simulink model "vehicle_dynamics"  (R2023a)
settings: Solver=FixedStepAuto  StartTime=0.0  StopTime=10.0  MaxStep=1e-3  RelTol=1e-3  EnableMultiTasking=on
undefined symbols (not defined in the file): A, b_vkm, c_W, eta, f_R, g, iD_car, iG_car, m_F, m_vkm, m_Zu, p, p_L, r_dyn, r_stat, v_0
settings Model: Creator=Sascha  LastModifiedBy=Sascha
settings SolverCC: AlgebraicLoopSolver=TrustRegion
settings OptimizationCC: EnhancedBackFolding=on  PassReuseOutputArgsAs=Individual arguments  ZeroExternalMemoryAtStartup=off  ZeroInternalMemoryAtStartup=off  MaxStackSize=64  OptimizeBlockOrder=speed  DifferentSizesBufferReuse=on  OptimizationCustomize=off  EfficientTunableParamExpr=on
settings DebuggingCC: ParameterTunabilityLossMsg=error  UnconnectedInputMsg=warning  UnconnectedOutputMsg=warning  UnconnectedLineMsg=warning
settings HardwareCC: ProdBitPerPointer=32  ProdBitPerSizeT=32  ProdBitPerPtrDiffT=32  ProdLargestAtomicInteger=Long  ProdLargestAtomicFloat=Double  ProdWordSize=32  ProdLongLongMode=on  ProdHWDeviceType=ARM Compatible->ARM Cortex
settings ModelReferenceCC: EnableRefExpFcnMdlSchedulingChecks=on
settings SFSimCC: MATLABDynamicMemAlloc=off
settings RTWCC: Description=Embedded Coder  SystemTargetFile=ert.tlc  HardwareBoard=STM32F746G-Discovery  TemplateMakefile=ert_default_tmf  Toolchain=GNU Tools for ARM Embedded Processors  DLArmComputeVersion=19.05
settings CodeAppCC: ForceParamTrailComments=on  IgnoreCustomStorageClasses=off  OperatorAnnotations=on  SimulinkDataObjDesc=on  SFDataObjDesc=on  InsertBlockDesc=on
settings ERTTargetCC: ExtModeTransport=3  ExtModeStaticAlloc=on  ExtModeStaticAllocSize=5000  ExtModeMexFile=ext_xcp  ExtModeIntrfLevel=Level2 - Open

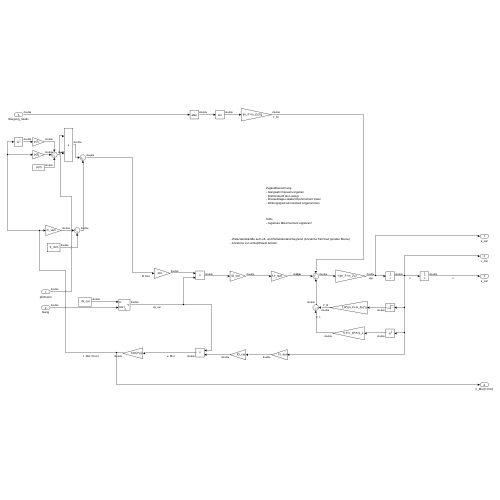
[thumbnail: Simulink's stored preview of the top-level diagram]
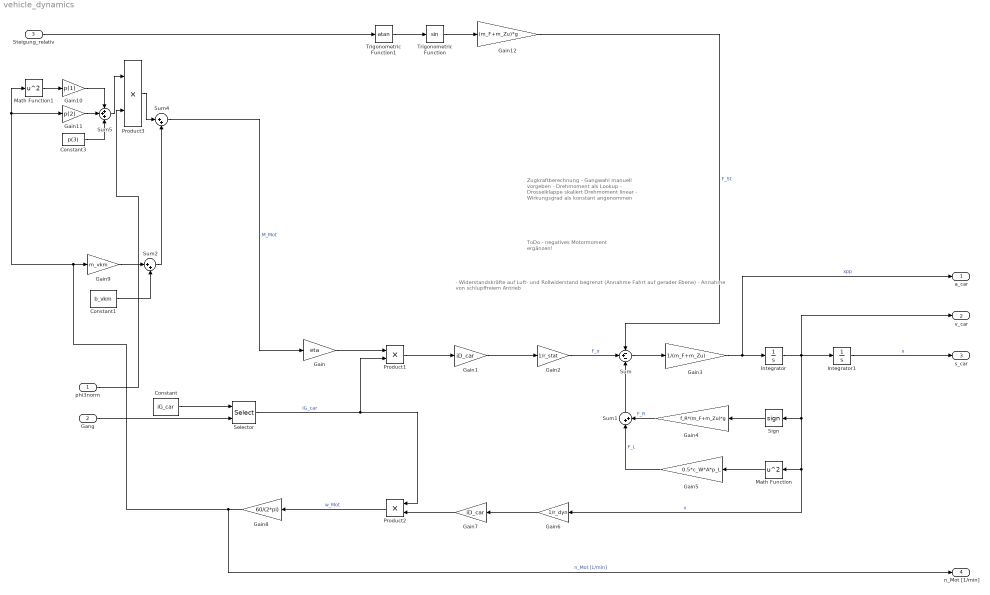
== system vehicle_dynamics ==
  note: Zugkraftberechnung
      | - Gangwahl manuell vorgeben
      | - Drehmoment als Lookup
      | - Drosselklappe skaliert Drehmoment linear
      | - Wirkungsgrad als konstant angenommen
  note: ToDo
      | - negatives Motormoment ergänzen!
  note: - Widerstandskräfte auf Luft- und Rollwiderstand begrenzt (Annahme Fahrt auf gerader Ebene)
      | - Annahme von schlupffreiem Antrieb
  phi3norm : Inport
  Gang : Inport  Port=2
  Steigung_relativ : Inport  Port=3
  Constant : Constant  Value=iG_car
  Constant1 : Constant  Value=b_vkm
  Constant3 : Constant  Value=p(3)
  Gain : Gain  Gain=eta
  Gain1 : Gain  Gain=iD_car
  Gain10 : Gain  Gain=p(1)
  Gain11 : Gain  Gain=p(2)
  Gain12 : Gain  Gain=(m_F+m_Zu)*g
  Gain2 : Gain  Gain=1/r_stat
  Gain3 : Gain  Gain=1/(m_F+m_Zu)
  Gain4 : Gain  Gain=f_R*(m_F+m_Zu)*g
  Gain5 : Gain  Gain=0.5*c_W*A*p_L
  Gain6 : Gain  Gain=1/r_dyn
  Gain7 : Gain  Gain=iD_car
  Gain8 : Gain  Gain=60/(2*pi)
  Gain9 : Gain  Gain=m_vkm
  Integrator : Integrator  InitialCondition=v_0
  Integrator1 : Integrator
  Math Function : Math  Operator=square
  Math Function1 : Math  Operator=square
  Product1 : Product
  Product2 : Product
  Product3 : Product
  Selector : Selector  IndexMode=Zero-based  InputPortWidth=6  IndexOptions=Index vector (port)  Indices=[1 3]  OutputSizes=1
  Sign : Signum
  Sum : Sum  Inputs=-+-
  Sum1 : Sum  Inputs=|++
  Sum2 : Sum  Inputs=|++
  Sum4 : Sum  Inputs=|++
  Sum5 : Sum  Inputs=+++
  Trigonometric Function : Trigonometry
  Trigonometric Function1 : Trigonometry  Operator=atan
  a_car : Outport
  v_car : Outport  Port=2
  s_car : Outport  Port=3
  n_Mot [1/min] : Outport  Port=4
  wires:
  Gain4/1 -> Sum1/2  "F_R"
  Gain3/1 -> a_car/1, Integrator/1  "xpp"
  Gain2/1 -> Sum/2  "F_x"
  Sum1/1 -> Sum/3
  Product2/1 -> Gain8/1  "w_Mot"
  Math Function/1 -> Gain5/1
  Sum/1 -> Gain3/1
  Gain1/1 -> Gain2/1
  Gain/1 -> Product1/1
  Selector/1 -> Product2/1, Product1/2  "iG_car"
  Product1/1 -> Gain1/1
  Constant/1 -> Selector/1
  Integrator1/1 -> s_car/1  "x"
  Gain6/1 -> Gain7/1
  Integrator/1 -> v_car/1, Gain6/1, Math Function/1, Sign/1, Integrator1/1  "v"
  Gain7/1 -> Product2/2
  Sign/1 -> Gain4/1
  Sum4/1 -> Gain/1  "M_Mot"
  Gain5/1 -> Sum1/1  "F_L"
  Gain8/1 -> n_Mot [1/min]/1, Gain9/1, Gain11/1, Math Function1/1  "n_Mot [1/min]"
  Gang/1 -> Selector/2
  phi3norm/1 -> Product3/2
  Constant1/1 -> Sum2/2
  Gain9/1 -> Sum2/1
  Sum2/1 -> Sum4/2
  Sum5/1 -> Product3/1
  Math Function1/1 -> Gain10/1
  Gain10/1 -> Sum5/1
  Gain11/1 -> Sum5/2
  Constant3/1 -> Sum5/3
  Product3/1 -> Sum4/1
  Gain12/1 -> Sum/1  "F_St"
  Trigonometric Function/1 -> Gain12/1
  Trigonometric Function1/1 -> Trigonometric Function/1
  Steigung_relativ/1 -> Trigonometric Function1/1
